simulink model "Hierarchy2"  (Simulink 8.7)
settings: Solver=ode45  StartTime=0.0  StopTime=10.0  RelTol=1e-3
settings Model: Creator=scaife  LastModifiedBy=bourbouh  ExtModeAutoUpdateStatusClock=off
settings DataIOCC: SignalLoggingSaveFormat=ModelDataLogs  SignalLoggingName=sigsOut
settings DebuggingCC: SaveWithParameterizedLinksMsg=none  SignalResolutionControl=TryResolveAllWithWarning  MultiTaskDSMMsg=warning  MultiTaskCondExecSysMsg=none
settings HardwareCC: TargetBitPerLong=64  TargetBitPerPointer=64  TargetLongLongMode=on  TargetIntDivRoundTo=Zero  TargetEndianess=LittleEndian  TargetWordSize=64  TargetHWDeviceType=MATLAB Host  ProdEqTarget=off
settings SFSimCC: SimParseCustomCode=off
settings GRTTargetCC: GeneratePreprocessorConditionals=Use local settings  CombineOutputUpdateFcns=off  GRTInterface=on

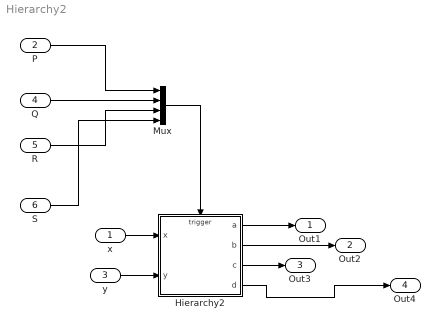
== system Hierarchy2 ==
  x : Inport
  P : Inport  Port=2
  y : Inport  Port=3
  Q : Inport  Port=4
  R : Inport  Port=5
  S : Inport  Port=6
  Hierarchy2 : Stateflow chart  TreatAsAtomicUnit=on
  Mux : Mux
  Out1 : Outport
  Out2 : Outport  Port=2
  Out3 : Outport  Port=3
  Out4 : Outport  Port=4
  wires:
  Hierarchy2/1(a) -> Out1/1
  Hierarchy2/2(b) -> Out2/1
  Hierarchy2/3(c) -> Out3/1
  Hierarchy2/4(d) -> Out4/1
  Mux/1 -> Hierarchy2/Trigger
  P/1 -> Mux/1
  Q/1 -> Mux/2
  R/1 -> Mux/3
  S/1 -> Mux/4
  x/1 -> Hierarchy2/1(x)
  y/1 -> Hierarchy2/2(y)

== stateflow chart Hierarchy2 ==
  state A
    state A1
      state A1a/
        en:a=x+1
        state A1aA
          state A1aA2
            state A1Aa2a
            state A1aA2b
            (default) -> A1Aa2a
            A1Aa2a -> A1aA2b : S
            A1aA2b -> A1Aa2a : S
          state A1aA1
            state A1aA1a
            state A1aA1b
            (default) -> A1aA1a
            A1aA1a -> A1aA1b : S
            A1aA1b -> A1aA1a : S
          (default) -> A1aA1
          A1aA1 -> A1aA2 : R
          A1aA2 -> A1aA1 : R
        (default) -> A1aA
      state A1b/
        en:a=x+2
        state A3aA
          state A3aA2
            state A3Aa2a
            state A3aA2b
            (default) -> A3Aa2a
            A3Aa2a -> A3aA2b : S
            A3aA2b -> A3Aa2a : S
          state A3aA1
            state A3aA1a
            state A3aA1b
            (default) -> A3aA1a
            A3aA1a -> A3aA1b : S
            A3aA1b -> A3aA1a : S
          (default) -> A3aA1
          A3aA1 -> A3aA2 : R
          A3aA2 -> A3aA1 : R
        (default) -> A3aA
      (default) -> A1a
      A1a -> A1b : Q
      A1b -> A1a : Q
    state A2
      state A2a/
        en:a=x+3
        state A2aA
          state A2aA2
            state A2Aa2a
            state A2aA2b
            (default) -> A2Aa2a
            A2Aa2a -> A2aA2b : S
            A2aA2b -> A2Aa2a : S
          state A2aA1
            state A2aA1a
            state A2aA1b
            (default) -> A2aA1a
            A2aA1a -> A2aA1b : S
            A2aA1b -> A2aA1a : S
          (default) -> A2aA1
          A2aA1 -> A2aA2 : R
          A2aA2 -> A2aA1 : R
        (default) -> A2aA
      state A2b/
        en:a=x+4
        state A4aA
          state A4aA2
            state A4Aa2a
            state A4aA2b
            (default) -> A4Aa2a
            A4Aa2a -> A4aA2b : S
            A4aA2b -> A4Aa2a : S
          state A4aA1
            state A4aA1a
            state A4aA1b
            (default) -> A4aA1a
            A4aA1a -> A4aA1b : S
            A4aA1b -> A4aA1a : S
          (default) -> A4aA1
          A4aA1 -> A4aA2 : R
          A4aA2 -> A4aA1 : R
        (default) -> A4aA
      (default) -> A2a
      A2a -> A2b : Q
      A2b -> A2a : Q
    (default) -> A1
    A1 -> A2 : P
    A2 -> A1 : P
  (default) -> A
  data: a output int32; b output int32; c output int32; d output int32; x input int32; y input int32
  events: P input EITHER_EDGE_EVENT; Q input EITHER_EDGE_EVENT; R input EITHER_EDGE_EVENT; S input EITHER_EDGE_EVENT
